simulink library "Electrical_to_Mechanical_gen"  (R2016a)
settings: Solver=ode45  StartTime=0.0  StopTime=10.0  RelTol=1e-3
undefined symbols (not defined in the file): API1dcac_efficiency, API2dcac_efficiency, API3dcac_efficiency, APIdcac_efficiency, aux_power_state, auxEmot_inertia, auxEmot_nTab_3rdD, auxEmot_power, auxEmot_pwrAC, auxEmot_Tau, auxEmot_trqTab_2ndD, auxEmot_vltTab_1stD, AWR_InvStError, DiscIntNeverNeededParam, drvEmot_emot_Cth_rotor, drvEmot_emot_Cth_stator, drvEmot_emot_dtrqEmotNeg, drvEmot_emot_dtrqEmotPtv, drvEmot_emot_inv_pwrLoss, drvEmot_emot_mot_pwrLoss, drvEmot_emot_Rth_rotor_oil, drvEmot_emot_Rth_stator_oil, drvEmot_emot_Rth_stator_rotor, drvEmot_emot_Trotor_init, drvEmot_emot_trqMaxRow, drvEmot_emot_trqMinRow, drvEmot_emot_Tstator_init, drvEmot_inv_Cth_cooling_plate, drvEmot_inv_Cth_diode, drvEmot_inv_Cth_IGBT, drvEmot_inv_n_IGBT_per_Switch, drvEmot_inv_Rth_cooling_plate_coolant, drvEmot_inv_Rth_PS_cooling_plate, drvEmot_inv_Tplate_init, drvEmot_inv_Tpowerstack_init, drvEmot_RefTqeMOT, emot_AcCmprFront_inertia, emot_AcCmprFront_nTab_3rdD, emot_AcCmprFront_pwrAC, emot_AcCmprFront_Tau, emot_AcCmprFront_trqTab_2ndD, emot_AcCmprFront_vltTab_1stD, emot_AcCmprRear_inertia, emot_AcCmprRear_nTab_3rdD, emot_AcCmprRear_pwrAC, emot_AcCmprRear_Tau, emot_AcCmprRear_trqTab_2ndD, emot_AcCmprRear_vltTab_1stD, emot_AirCmpr_inertia, emot_AirCmpr_nTab_3rdD, emot_AirCmpr_pwrAC, emot_AirCmpr_Tau, emot_AirCmpr_trqTab_2ndD, emot_AirCmpr_vltTab_1stD, emot_aircomp_power, FirstDrivenAxle_FirstDrivenAxleNoOfEmot, SecondDrivenAxle_SecondDrivenAxleNoOfEmot
libraries: Electrical_to_Mechanical_gen x4, simulink x4
(part 2 of 2)

== system Electrical_to_Mechanical_gen/EDB_DriveEmot/Emot2_3 ==
  hvs_emot_Emot2_angVel : Inport
  voltBatHV2 : Inport  Port=2
  trqEmotDesPhy2 : Inport  Port=3
  emot_CMD2 : Inport  Port=4
  voltBatHV3 : Inport  Port=5
  trqEmotDesPhy3 : Inport  Port=6
  emot_CMD3 : Inport  Port=7
  hvs_drvEmot2Oil_Temperature : Inport  Port=8
  inv_coolant_temperature : Inport  Port=9
  Emot2_Selection : Inport  Port=10
  Emot3_Selection : Inport  Port=11
  hvs_emot_Emot3_angVel : Inport  Port=12
  hvs_drvEmot3Oil_Temperature : Inport  Port=13
  Bus Creator1 : BusCreator  Inputs=12
  Bus Creator2 : BusCreator  Inputs=12
  Bus Creator3 : BusCreator  Inputs=2
  e-Motor2 : Electrical_to_Mechanical_gen/e-Motor  SystemSampleTime=-1
  e-Motor3 : Electrical_to_Mechanical_gen/e-Motor  SystemSampleTime=-1
  emot2_3B : Outport
  wires:
  e-Motor3/12 -> Bus Creator2/12
  e-Motor3/11 -> Bus Creator2/11
  e-Motor2/12 -> Bus Creator1/12
  e-Motor2/11 -> Bus Creator1/11
  e-Motor3/10 -> Bus Creator2/10
  e-Motor2/10 -> Bus Creator1/10
  hvs_drvEmot3Oil_Temperature/1 -> e-Motor3/5
  Emot3_Selection/1 -> e-Motor3/Enable
  Emot2_Selection/1 -> e-Motor2/Enable
  emot_CMD3/1 -> e-Motor3/4
  emot_CMD2/1 -> e-Motor2/4
  e-Motor3/5 -> Bus Creator2/5
  e-Motor3/4 -> Bus Creator2/4
  e-Motor3/3 -> Bus Creator2/3
  e-Motor3/2 -> Bus Creator2/2
  e-Motor3/1 -> Bus Creator2/1
  e-Motor2/5 -> Bus Creator1/5
  e-Motor2/2 -> Bus Creator1/2
  e-Motor2/1 -> Bus Creator1/1
  e-Motor2/4 -> Bus Creator1/4
  e-Motor2/3 -> Bus Creator1/3
  hvs_emot_Emot2_angVel/1 -> e-Motor2/1
  trqEmotDesPhy2/1 -> e-Motor2/3
  voltBatHV2/1 -> e-Motor2/2
  hvs_emot_Emot3_angVel/1 -> e-Motor3/1
  voltBatHV3/1 -> e-Motor3/2
  Bus Creator1/1 -> Bus Creator3/1  "emot2B"
  Bus Creator2/1 -> Bus Creator3/2  "emot3B"
  trqEmotDesPhy3/1 -> e-Motor3/3
  Bus Creator3/1 -> emot2_3B/1  "emot2_3B"
  hvs_drvEmot2Oil_Temperature/1 -> e-Motor2/5
  inv_coolant_temperature/1 -> e-Motor3/6, e-Motor2/6
  e-Motor3/7 -> Bus Creator2/7
  e-Motor3/6 -> Bus Creator2/6
  e-Motor3/8 -> Bus Creator2/8
  e-Motor3/9 -> Bus Creator2/9
  e-Motor2/6 -> Bus Creator1/6
  e-Motor2/7 -> Bus Creator1/7
  e-Motor2/9 -> Bus Creator1/9
  e-Motor2/8 -> Bus Creator1/8

== system Electrical_to_Mechanical_gen/EDB_DriveEmot/MotorSelection ==
  MidAxle : Constant  Value=FirstDrivenAxle_FirstDrivenAxleNoOfEmot
  RearAxle : Constant  Value=SecondDrivenAxle_SecondDrivenAxleNoOfEmot
  Truth Table : Truth Table  TreatAsAtomicUnit=on
  Emot1_Selection : Outport
  Emot2_Selection : Outport  Port=2
  Emot3_Selection : Outport  Port=3
  Emot4_Selection : Outport  Port=4
  wires:
  Truth Table/4(y4) -> Emot4_Selection/1
  Truth Table/3(y3) -> Emot3_Selection/1
  Truth Table/2(y2) -> Emot2_Selection/1
  Truth Table/1(y1) -> Emot1_Selection/1
  RearAxle/1 -> Truth Table/2(u2)
  MidAxle/1 -> Truth Table/1(u1)

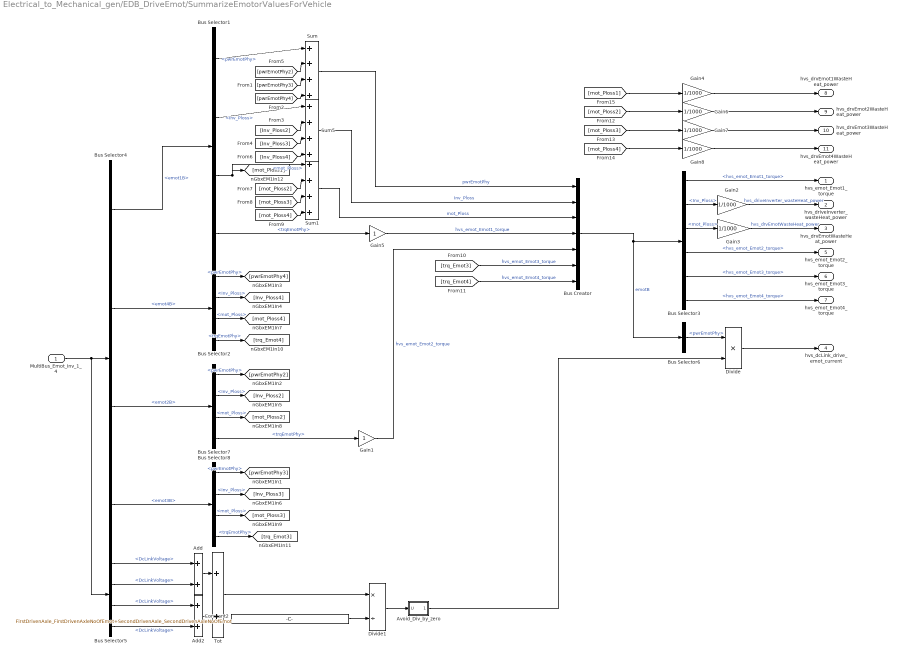
== system Electrical_to_Mechanical_gen/EDB_DriveEmot/SummarizeEmotorValuesForVehicle ==
  MultiBus_Emot_Inv_1_4 : Inport
  Add : Sum
  Add2 : Sum
  Avoid_Div_by_zero : Subsystem
  Bus Creator : BusCreator  Inputs=7
  Bus Selector{1..2,7..8} (4 alike) : BusSelector  OutputSignals=pwrEmotPhy,Inv_Ploss,mot_Ploss,trqEmotPhy
  Bus Selector3 : BusSelector  OutputSignals=hvs_emot_Emot1_torque,Inv_Ploss,mot_Ploss,hvs_emot_Emot2_torque,hvs_emot_Emot3_torque,hvs_emot_Emot4_torque
  Bus Selector4 : BusSelector  OutputSignals=emot1_4B.emot1B,emot1_4B.emot4B,emot2_3B.emot2B,emot2_3B.emot3B
  Bus Selector5 : BusSelector  OutputSignals=emot1_4B.emot1B.DcLinkVoltage,emot1_4B.emot4B.DcLinkVoltage,emot2_3B.emot2B.DcLinkVoltage,emot2_3B.emot3B.DcLinkVoltage
  Bus Selector6 : BusSelector  OutputSignals=pwrEmotPhy
  Constant2 : Constant  Value=FirstDrivenAxle_FirstDrivenAxleNoOfEmot+SecondDrivenAxle_SecondDrivenAxleNoOfEmot
  Divide : Product  Inputs=**
  Divide1 : Product  Inputs=*/
  Gain1 : Gain
  Gain{2..4,6..8} (6 alike) : Gain  Gain=1/1000
  Gain5 : Gain
  Sum : Sum  Inputs=|++++
  Sum1 : Sum  Inputs=|++++
  Sum5 : Sum  Inputs=|++++
  Tot : Sum
  hvs_emot_Emot1_torque : Outport
  hvs_driveInverter_wasteHeat_power : Outport  Port=2
  hvs_drvEmotWasteHeat_power : Outport  Port=3
  hvs_dcLink_drive_emot_current : Outport  Port=4
  hvs_emot_Emot2_torque : Outport  Port=5
  hvs_emot_Emot3_torque : Outport  Port=6
  hvs_emot_Emot4_torque : Outport  Port=7
  hvs_drvEmot1WasteHeat_power : Outport  Port=8
  hvs_drvEmot2WasteHeat_power : Outport  Port=9
  hvs_drvEmot3WasteHeat_power : Outport  Port=10
  hvs_drvEmot4WasteHeat_power : Outport  Port=11
  wires:
  Gain8/1 -> hvs_drvEmot4WasteHeat_power/1
  Gain7/1 -> hvs_drvEmot3WasteHeat_power/1
  Gain6/1 -> hvs_drvEmot2WasteHeat_power/1
  Gain4/1 -> hvs_drvEmot1WasteHeat_power/1
  [mot_Ploss4] -> Gain8/1
  [mot_Ploss3] -> Gain7/1
  [mot_Ploss2] -> Gain6/1
  [mot_Ploss1] -> Gain4/1
  Bus Selector3/6 -> hvs_emot_Emot4_torque/1  "<hvs_emot_Emot4_torque>"
  Bus Selector3/5 -> hvs_emot_Emot3_torque/1  "<hvs_emot_Emot3_torque>"
  Bus Selector3/4 -> hvs_emot_Emot2_torque/1  "<hvs_emot_Emot2_torque>"
  Bus Selector3/1 -> hvs_emot_Emot1_torque/1  "<hvs_emot_Emot1_torque>"
  [trq_Emot4] -> Bus Creator/7  "hvs_emot_Emot4_torque"
  [trq_Emot3] -> Bus Creator/6  "hvs_emot_Emot3_torque"
  Bus Selector2/4 -> [trq_Emot4]  "<trqEmotPhy>"
  Tot/1 -> Divide1/1
  Constant2/1 -> Divide1/2
  Add2/1 -> Tot/2
  Bus Selector5/4 -> Add2/2  "<DcLinkVoltage>"
  Bus Selector5/3 -> Add2/1  "<DcLinkVoltage>"
  Gain1/1 -> Bus Creator/5  "hvs_emot_Emot2_torque"
  Bus Selector8/4 -> [trq_Emot3]  "<trqEmotPhy>"
  Bus Selector7/4 -> Gain1/1  "<trqEmotPhy>"
  [mot_Ploss4] -> Sum1/4
  [mot_Ploss3] -> Sum1/3
  [mot_Ploss2] -> Sum1/2
  Bus Selector8/3 -> [mot_Ploss3]  "<mot_Ploss>"
  Bus Selector7/3 -> [mot_Ploss2]  "<mot_Ploss>"
  Bus Selector8/2 -> [Inv_Ploss3]  "<Inv_Ploss>"
  Bus Selector7/2 -> [Inv_Ploss2]  "<Inv_Ploss>"
  [Inv_Ploss4] -> Sum5/4
  [Inv_Ploss3] -> Sum5/3
  [Inv_Ploss2] -> Sum5/2
  [pwrEmotPhy4] -> Sum/4
  [pwrEmotPhy3] -> Sum/3
  [pwrEmotPhy2] -> Sum/2
  Bus Selector2/1 -> [pwrEmotPhy4]  "<pwrEmotPhy>"
  Bus Selector8/1 -> [pwrEmotPhy3]  "<pwrEmotPhy>"
  Bus Selector7/1 -> [pwrEmotPhy2]  "<pwrEmotPhy>"
  Bus Selector4/3 -> Bus Selector7/1  "<emot2B>"
  Bus Selector4/4 -> Bus Selector8/1  "<emot3B>"
  Gain3/1 -> hvs_drvEmotWasteHeat_power/1  "hvs_drvEmotWasteHeat_power"
  Bus Selector3/3 -> Gain3/1  "<mot_Ploss>"
  Gain2/1 -> hvs_driveInverter_wasteHeat_power/1  "hvs_driveInverter_wasteHeat_power"
  Bus Selector3/2 -> Gain2/1  "<Inv_Ploss>"
  Divide/1 -> hvs_dcLink_drive_emot_current/1
  Avoid_Div_by_zero/1(1/U) -> Divide/2
  Bus Selector6/1 -> Divide/1  "<pwrEmotPhy>"
  Divide1/1 -> Avoid_Div_by_zero/1(U)
  Add/1 -> Tot/1
  Bus Selector5/2 -> Add/2  "<DcLinkVoltage>"
  Bus Selector5/1 -> Add/1  "<DcLinkVoltage>"
  Bus Creator/1 -> Bus Selector6/1, Bus Selector3/1  "emotB"
  MultiBus_Emot_Inv_1_4/1 -> Bus Selector4/1, Bus Selector5/1
  Bus Selector4/1 -> Bus Selector1/1  "<emot1B>"
  Bus Selector4/2 -> Bus Selector2/1  "<emot4B>"
  Bus Selector1/1 -> Sum/1  "<pwrEmotPhy>"
  Bus Selector1/2 -> Sum5/1  "<Inv_Ploss>"
  Bus Selector2/2 -> [Inv_Ploss4]  "<Inv_Ploss>"
  Bus Selector1/3 -> Sum1/1, [mot_Ploss1]  "<mot_Ploss>"
  Bus Selector2/3 -> [mot_Ploss4]  "<mot_Ploss>"
  Bus Selector1/4 -> Gain5/1  "<trqEmotPhy>"
  Sum/1 -> Bus Creator/1  "pwrEmotPhy"
  Sum5/1 -> Bus Creator/2  "Inv_Ploss"
  Sum1/1 -> Bus Creator/3  "mot_Ploss"
  Gain5/1 -> Bus Creator/4  "hvs_emot_Emot1_torque"

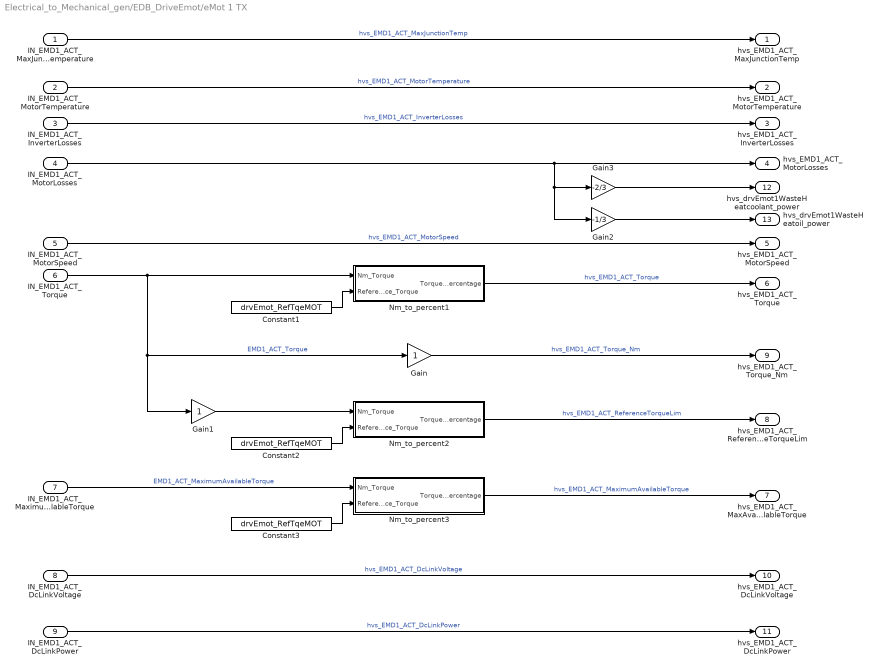
== system Electrical_to_Mechanical_gen/EDB_DriveEmot/eMot 1 TX ==
  IN_EMD1_ACT_MaxJunctionTemperature : Inport
  IN_EMD1_ACT_MotorTemperature : Inport  Port=2
  IN_EMD1_ACT_InverterLosses : Inport  Port=3
  IN_EMD1_ACT_MotorLosses : Inport  Port=4
  IN_EMD1_ACT_MotorSpeed : Inport  Port=5
  IN_EMD1_ACT_Torque : Inport  Port=6
  IN_EMD1_ACT_MaximumAvailableTorque : Inport  Port=7
  IN_EMD1_ACT_DcLinkVoltage : Inport  Port=8
  IN_EMD1_ACT_DcLinkPower : Inport  Port=9
  Constant1 : Constant  Value=drvEmot_RefTqeMOT
  Constant2 : Constant  Value=drvEmot_RefTqeMOT
  Constant3 : Constant  Value=drvEmot_RefTqeMOT
  Gain : Gain
  Gain1 : Gain
  Gain2 : Gain  Gain=-1/3
  Gain3 : Gain  Gain=-2/3
  Nm_to_percent1 : Subsystem
  Nm_to_percent2 : Subsystem
  Nm_to_percent3 : Subsystem
  hvs_EMD1_ACT_MaxJunctionTemp : Outport
  hvs_EMD1_ACT_MotorTemperature : Outport  Port=2
  hvs_EMD1_ACT_InverterLosses : Outport  Port=3
  hvs_EMD1_ACT_MotorLosses : Outport  Port=4
  hvs_EMD1_ACT_MotorSpeed : Outport  Port=5
  hvs_EMD1_ACT_Torque : Outport  Port=6
  hvs_EMD1_ACT_MaxAvailableTorque : Outport  Port=7
  hvs_EMD1_ACT_ReferenceTorqueLim : Outport  Port=8
  hvs_EMD1_ACT_Torque_Nm : Outport  Port=9
  hvs_EMD1_ACT_DcLinkVoltage : Outport  Port=10
  hvs_EMD1_ACT_DcLinkPower : Outport  Port=11
  hvs_drvEmot1WasteHeatcoolant_power : Outport  Port=12
  hvs_drvEmot1WasteHeatoil_power : Outport  Port=13
  wires:
  IN_EMD1_ACT_DcLinkVoltage/1 -> hvs_EMD1_ACT_DcLinkVoltage/1  "hvs_EMD1_ACT_DcLinkVoltage"
  IN_EMD1_ACT_DcLinkPower/1 -> hvs_EMD1_ACT_DcLinkPower/1  "hvs_EMD1_ACT_DcLinkPower"
  Nm_to_percent2/1(Torque_Percentage) -> hvs_EMD1_ACT_ReferenceTorqueLim/1  "hvs_EMD1_ACT_ReferenceTorqueLim"
  Constant2/1 -> Nm_to_percent2/2(Reference_Torque)
  Gain1/1 -> Nm_to_percent2/1(Nm_Torque)
  Gain/1 -> hvs_EMD1_ACT_Torque_Nm/1  "hvs_EMD1_ACT_Torque_Nm"
  Constant1/1 -> Nm_to_percent1/2(Reference_Torque)
  IN_EMD1_ACT_Torque/1 -> Nm_to_percent1/1(Nm_Torque), Gain1/1, Gain/1  "EMD1_ACT_Torque"
  IN_EMD1_ACT_MaximumAvailableTorque/1 -> Nm_to_percent3/1(Nm_Torque)  "EMD1_ACT_MaximumAvailableTorque"
  Constant3/1 -> Nm_to_percent3/2(Reference_Torque)
  Nm_to_percent1/1(Torque_Percentage) -> hvs_EMD1_ACT_Torque/1  "hvs_EMD1_ACT_Torque"
  Nm_to_percent3/1(Torque_Percentage) -> hvs_EMD1_ACT_MaxAvailableTorque/1  "hvs_EMD1_ACT_MaximumAvailableTorque"
  IN_EMD1_ACT_InverterLosses/1 -> hvs_EMD1_ACT_InverterLosses/1  "hvs_EMD1_ACT_InverterLosses"
  IN_EMD1_ACT_MotorTemperature/1 -> hvs_EMD1_ACT_MotorTemperature/1  "hvs_EMD1_ACT_MotorTemperature"
  IN_EMD1_ACT_MaxJunctionTemperature/1 -> hvs_EMD1_ACT_MaxJunctionTemp/1  "hvs_EMD1_ACT_MaxJunctionTemp"
  IN_EMD1_ACT_MotorSpeed/1 -> hvs_EMD1_ACT_MotorSpeed/1  "hvs_EMD1_ACT_MotorSpeed"
  IN_EMD1_ACT_MotorLosses/1 -> Gain3/1, Gain2/1, hvs_EMD1_ACT_MotorLosses/1
  Gain2/1 -> hvs_drvEmot1WasteHeatoil_power/1
  Gain3/1 -> hvs_drvEmot1WasteHeatcoolant_power/1

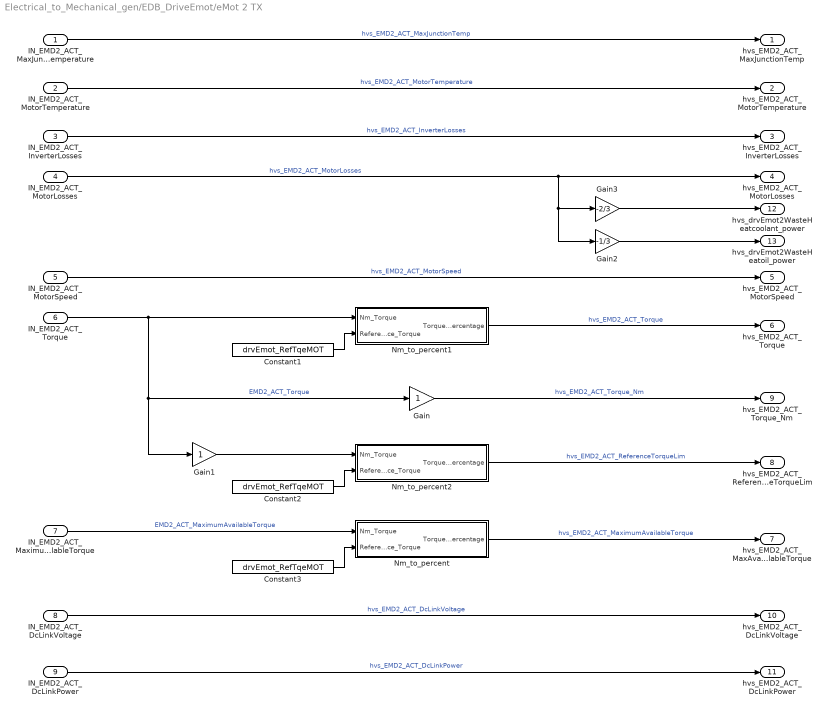
== system Electrical_to_Mechanical_gen/EDB_DriveEmot/eMot 2 TX ==
  IN_EMD2_ACT_MaxJunctionTemperature : Inport
  IN_EMD2_ACT_MotorTemperature : Inport  Port=2
  IN_EMD2_ACT_InverterLosses : Inport  Port=3
  IN_EMD2_ACT_MotorLosses : Inport  Port=4
  IN_EMD2_ACT_MotorSpeed : Inport  Port=5
  IN_EMD2_ACT_Torque : Inport  Port=6
  IN_EMD2_ACT_MaximumAvailableTorque : Inport  Port=7
  IN_EMD2_ACT_DcLinkVoltage : Inport  Port=8
  IN_EMD2_ACT_DcLinkPower : Inport  Port=9
  Constant1 : Constant  Value=drvEmot_RefTqeMOT
  Constant2 : Constant  Value=drvEmot_RefTqeMOT
  Constant3 : Constant  Value=drvEmot_RefTqeMOT
  Gain : Gain
  Gain1 : Gain
  Gain2 : Gain  Gain=-1/3
  Gain3 : Gain  Gain=-2/3
  Nm_to_percent : Subsystem
  Nm_to_percent1 : Subsystem
  Nm_to_percent2 : Subsystem
  hvs_EMD2_ACT_MaxJunctionTemp : Outport
  hvs_EMD2_ACT_MotorTemperature : Outport  Port=2
  hvs_EMD2_ACT_InverterLosses : Outport  Port=3
  hvs_EMD2_ACT_MotorLosses : Outport  Port=4
  hvs_EMD2_ACT_MotorSpeed : Outport  Port=5
  hvs_EMD2_ACT_Torque : Outport  Port=6
  hvs_EMD2_ACT_MaxAvailableTorque : Outport  Port=7
  hvs_EMD2_ACT_ReferenceTorqueLim : Outport  Port=8
  hvs_EMD2_ACT_Torque_Nm : Outport  Port=9
  hvs_EMD2_ACT_DcLinkVoltage : Outport  Port=10
  hvs_EMD2_ACT_DcLinkPower : Outport  Port=11
  hvs_drvEmot2WasteHeatcoolant_power : Outport  Port=12
  hvs_drvEmot2WasteHeatoil_power : Outport  Port=13
  wires:
  IN_EMD2_ACT_DcLinkPower/1 -> hvs_EMD2_ACT_DcLinkPower/1  "hvs_EMD2_ACT_DcLinkPower"
  IN_EMD2_ACT_DcLinkVoltage/1 -> hvs_EMD2_ACT_DcLinkVoltage/1  "hvs_EMD2_ACT_DcLinkVoltage"
  Nm_to_percent2/1(Torque_Percentage) -> hvs_EMD2_ACT_ReferenceTorqueLim/1  "hvs_EMD2_ACT_ReferenceTorqueLim"
  Constant2/1 -> Nm_to_percent2/2(Reference_Torque)
  Gain1/1 -> Nm_to_percent2/1(Nm_Torque)
  Gain/1 -> hvs_EMD2_ACT_Torque_Nm/1  "hvs_EMD2_ACT_Torque_Nm"
  Constant1/1 -> Nm_to_percent1/2(Reference_Torque)
  IN_EMD2_ACT_Torque/1 -> Nm_to_percent1/1(Nm_Torque), Gain1/1, Gain/1  "EMD2_ACT_Torque"
  IN_EMD2_ACT_MaximumAvailableTorque/1 -> Nm_to_percent/1(Nm_Torque)  "EMD2_ACT_MaximumAvailableTorque"
  Constant3/1 -> Nm_to_percent/2(Reference_Torque)
  IN_EMD2_ACT_MotorLosses/1 -> Gain3/1, Gain2/1, hvs_EMD2_ACT_MotorLosses/1  "hvs_EMD2_ACT_MotorLosses"
  IN_EMD2_ACT_InverterLosses/1 -> hvs_EMD2_ACT_InverterLosses/1  "hvs_EMD2_ACT_InverterLosses"
  IN_EMD2_ACT_MotorTemperature/1 -> hvs_EMD2_ACT_MotorTemperature/1  "hvs_EMD2_ACT_MotorTemperature"
  IN_EMD2_ACT_MaxJunctionTemperature/1 -> hvs_EMD2_ACT_MaxJunctionTemp/1  "hvs_EMD2_ACT_MaxJunctionTemp"
  IN_EMD2_ACT_MotorSpeed/1 -> hvs_EMD2_ACT_MotorSpeed/1  "hvs_EMD2_ACT_MotorSpeed"
  Nm_to_percent1/1(Torque_Percentage) -> hvs_EMD2_ACT_Torque/1  "hvs_EMD2_ACT_Torque"
  Nm_to_percent/1(Torque_Percentage) -> hvs_EMD2_ACT_MaxAvailableTorque/1  "hvs_EMD2_ACT_MaximumAvailableTorque"
  Gain2/1 -> hvs_drvEmot2WasteHeatoil_power/1
  Gain3/1 -> hvs_drvEmot2WasteHeatcoolant_power/1

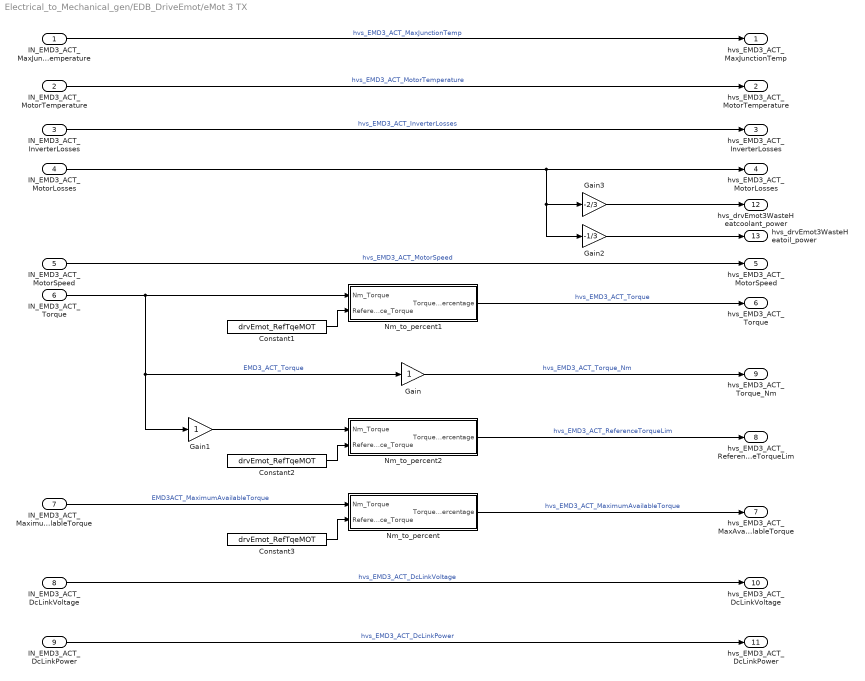
== system Electrical_to_Mechanical_gen/EDB_DriveEmot/eMot 3 TX ==
  IN_EMD3_ACT_MaxJunctionTemperature : Inport
  IN_EMD3_ACT_MotorTemperature : Inport  Port=2
  IN_EMD3_ACT_InverterLosses : Inport  Port=3
  IN_EMD3_ACT_MotorLosses : Inport  Port=4
  IN_EMD3_ACT_MotorSpeed : Inport  Port=5
  IN_EMD3_ACT_Torque : Inport  Port=6
  IN_EMD3_ACT_MaximumAvailableTorque : Inport  Port=7
  IN_EMD3_ACT_DcLinkVoltage : Inport  Port=8
  IN_EMD3_ACT_DcLinkPower : Inport  Port=9
  Constant1 : Constant  Value=drvEmot_RefTqeMOT
  Constant2 : Constant  Value=drvEmot_RefTqeMOT
  Constant3 : Constant  Value=drvEmot_RefTqeMOT
  Gain : Gain
  Gain1 : Gain
  Gain2 : Gain  Gain=-1/3
  Gain3 : Gain  Gain=-2/3
  Nm_to_percent : Subsystem
  Nm_to_percent1 : Subsystem
  Nm_to_percent2 : Subsystem
  hvs_EMD3_ACT_MaxJunctionTemp : Outport
  hvs_EMD3_ACT_MotorTemperature : Outport  Port=2
  hvs_EMD3_ACT_InverterLosses : Outport  Port=3
  hvs_EMD3_ACT_MotorLosses : Outport  Port=4
  hvs_EMD3_ACT_MotorSpeed : Outport  Port=5
  hvs_EMD3_ACT_Torque : Outport  Port=6
  hvs_EMD3_ACT_MaxAvailableTorque : Outport  Port=7
  hvs_EMD3_ACT_ReferenceTorqueLim : Outport  Port=8
  hvs_EMD3_ACT_Torque_Nm : Outport  Port=9
  hvs_EMD3_ACT_DcLinkVoltage : Outport  Port=10
  hvs_EMD3_ACT_DcLinkPower : Outport  Port=11
  hvs_drvEmot3WasteHeatcoolant_power : Outport  Port=12
  hvs_drvEmot3WasteHeatoil_power : Outport  Port=13
  wires:
  IN_EMD3_ACT_DcLinkPower/1 -> hvs_EMD3_ACT_DcLinkPower/1  "hvs_EMD3_ACT_DcLinkPower"
  IN_EMD3_ACT_DcLinkVoltage/1 -> hvs_EMD3_ACT_DcLinkVoltage/1  "hvs_EMD3_ACT_DcLinkVoltage"
  Nm_to_percent2/1(Torque_Percentage) -> hvs_EMD3_ACT_ReferenceTorqueLim/1  "hvs_EMD3_ACT_ReferenceTorqueLim"
  Constant2/1 -> Nm_to_percent2/2(Reference_Torque)
  Gain1/1 -> Nm_to_percent2/1(Nm_Torque)
  Gain/1 -> hvs_EMD3_ACT_Torque_Nm/1  "hvs_EMD3_ACT_Torque_Nm"
  Constant1/1 -> Nm_to_percent1/2(Reference_Torque)
  IN_EMD3_ACT_Torque/1 -> Nm_to_percent1/1(Nm_Torque), Gain1/1, Gain/1  "EMD3_ACT_Torque"
  IN_EMD3_ACT_MaximumAvailableTorque/1 -> Nm_to_percent/1(Nm_Torque)  "EMD3ACT_MaximumAvailableTorque"
  Constant3/1 -> Nm_to_percent/2(Reference_Torque)
  Nm_to_percent1/1(Torque_Percentage) -> hvs_EMD3_ACT_Torque/1  "hvs_EMD3_ACT_Torque"
  Nm_to_percent/1(Torque_Percentage) -> hvs_EMD3_ACT_MaxAvailableTorque/1  "hvs_EMD3_ACT_MaximumAvailableTorque"
  IN_EMD3_ACT_InverterLosses/1 -> hvs_EMD3_ACT_InverterLosses/1  "hvs_EMD3_ACT_InverterLosses"
  IN_EMD3_ACT_MaxJunctionTemperature/1 -> hvs_EMD3_ACT_MaxJunctionTemp/1  "hvs_EMD3_ACT_MaxJunctionTemp"
  IN_EMD3_ACT_MotorTemperature/1 -> hvs_EMD3_ACT_MotorTemperature/1  "hvs_EMD3_ACT_MotorTemperature"
  IN_EMD3_ACT_MotorSpeed/1 -> hvs_EMD3_ACT_MotorSpeed/1  "hvs_EMD3_ACT_MotorSpeed"
  IN_EMD3_ACT_MotorLosses/1 -> hvs_EMD3_ACT_MotorLosses/1, Gain3/1, Gain2/1
  Gain2/1 -> hvs_drvEmot3WasteHeatoil_power/1
  Gain3/1 -> hvs_drvEmot3WasteHeatcoolant_power/1

== system Electrical_to_Mechanical_gen/EDB_DriveEmot/eMot 4 TX ==
  IN_EMD4_ACT_MaxJunctionTemperature : Inport
  IN_EMD4_ACT_MotorTemperature : Inport  Port=2
  IN_EMD4_ACT_InverterLosses : Inport  Port=3
  IN_EMD4_ACT_MotorLosses : Inport  Port=4
  IN_EMD4_ACT_MotorSpeed : Inport  Port=5
  IN_EMD4_ACT_Torque : Inport  Port=6
  IN_EMD4_ACT_MaximumAvailableTorque : Inport  Port=7
  IN_EMD4_ACT_DcLinkVoltage : Inport  Port=8
  IN_EMD4_ACT_DcLinkPower : Inport  Port=9
  Constant1 : Constant  Value=drvEmot_RefTqeMOT
  Constant2 : Constant  Value=drvEmot_RefTqeMOT
  Constant3 : Constant  Value=drvEmot_RefTqeMOT
  Gain : Gain
  Gain1 : Gain
  Gain2 : Gain  Gain=-1/3
  Gain3 : Gain  Gain=-2/3
  Nm_to_percent1 : Subsystem
  Nm_to_percent2 : Subsystem
  Nm_to_percent3 : Subsystem
  hvs_EMD4_ACT_MaxJunctionTemperature : Outport
  hvs_EMD4_ACT_MotorTemperature : Outport  Port=2
  hvs_EMD4_ACT_InverterLosses : Outport  Port=3
  hvs_EMD4_ACT_MotorLosses : Outport  Port=4
  hvs_EMD4_ACT_MotorSpeed : Outport  Port=5
  hvs_EMD4_ACT_Torque : Outport  Port=6
  hvs_EMD4_ACT_MaxAvailableTorque : Outport  Port=7
  hvs_EMD4_ACT_ReferenceTorqueLim : Outport  Port=8
  hvs_EMD4_ACT_Torque_Nm : Outport  Port=9
  hvs_EMD4_ACT_DcLinkVoltage : Outport  Port=10
  hvs_EMD4_ACT_DcLinkPower : Outport  Port=11
  hvs_drvEmot4WasteHeatcoolant_power : Outport  Port=12
  hvs_drvEmot4WasteHeatoil_power : Outport  Port=13
  wires:
  IN_EMD4_ACT_DcLinkPower/1 -> hvs_EMD4_ACT_DcLinkPower/1  "IN_EMD4_ACT_DcLinkPower"
  IN_EMD4_ACT_DcLinkVoltage/1 -> hvs_EMD4_ACT_DcLinkVoltage/1  "hvs_EMD4_ACT_DcLinkVoltage"
  Nm_to_percent2/1(Torque_Percentage) -> hvs_EMD4_ACT_ReferenceTorqueLim/1  "hvs_EMD4_ACT_ReferenceTorqueLim"
  Constant2/1 -> Nm_to_percent2/2(Reference_Torque)
  Gain1/1 -> Nm_to_percent2/1(Nm_Torque)
  Gain/1 -> hvs_EMD4_ACT_Torque_Nm/1  "hvs_EMD4_ACT_Torque_Nm"
  Constant1/1 -> Nm_to_percent1/2(Reference_Torque)
  IN_EMD4_ACT_Torque/1 -> Nm_to_percent1/1(Nm_Torque), Gain1/1, Gain/1  "EMD4_ACT_Torque"
  IN_EMD4_ACT_MaximumAvailableTorque/1 -> Nm_to_percent3/1(Nm_Torque)  "EMD4_ACT_MaximumAvailableTorque"
  Constant3/1 -> Nm_to_percent3/2(Reference_Torque)
  Nm_to_percent1/1(Torque_Percentage) -> hvs_EMD4_ACT_Torque/1  "hvs_EMD4_ACT_Torque"
  Nm_to_percent3/1(Torque_Percentage) -> hvs_EMD4_ACT_MaxAvailableTorque/1  "hvs_EMD4_ACT_MaximumAvailableTorque"
  IN_EMD4_ACT_InverterLosses/1 -> hvs_EMD4_ACT_InverterLosses/1  "hvs_EMD4_ACT_InverterLosses"
  IN_EMD4_ACT_MotorTemperature/1 -> hvs_EMD4_ACT_MotorTemperature/1  "hvs_EMD4_ACT_MotorTemperature"
  IN_EMD4_ACT_MaxJunctionTemperature/1 -> hvs_EMD4_ACT_MaxJunctionTemperature/1  "hvs_EMD4_ACT_MaxJunctionTemperature"
  IN_EMD4_ACT_MotorSpeed/1 -> hvs_EMD4_ACT_MotorSpeed/1  "hvs_EMD4_ACT_MotorSpeed"
  IN_EMD4_ACT_MotorLosses/1 -> Gain3/1, Gain2/1, hvs_EMD4_ACT_MotorLosses/1
  Gain2/1 -> hvs_drvEmot4WasteHeatoil_power/1
  Gain3/1 -> hvs_drvEmot4WasteHeatcoolant_power/1

== system Electrical_to_Mechanical_gen/Emot AC Compressor Front/Avoid_Div_by_zero ==
  U : Inport
  Constant : Constant  Value=10^-6
  Divide : Product  Inputs=/*
  Math Function : Math  Operator=square  SaturateOnIntegerOverflow=on
  Sum : Sum  Inputs=++|
  1/U : Outport
  wires:
  Divide/1 -> 1/U/1
  Math Function/1 -> Divide/1
  Sum/1 -> Divide/2, Math Function/1
  Constant/1 -> Sum/1
  U/1 -> Sum/2

== system Electrical_to_Mechanical_gen/Emot AC Compressor Rear/Avoid_Div_by_zero ==
  U : Inport
  Constant : Constant  Value=10^-6
  Divide : Product  Inputs=/*
  Math Function : Math  Operator=square  SaturateOnIntegerOverflow=on
  Sum : Sum  Inputs=++|
  1/U : Outport
  wires:
  Divide/1 -> 1/U/1
  Math Function/1 -> Divide/1
  Sum/1 -> Divide/2, Math Function/1
  Constant/1 -> Sum/1
  U/1 -> Sum/2

== system Electrical_to_Mechanical_gen/Emot Air Compressor/Avoid_Div_by_zero ==
  U : Inport
  Constant : Constant  Value=10^-6
  Divide : Product  Inputs=/*
  Math Function : Math  Operator=square  SaturateOnIntegerOverflow=on
  Sum : Sum  Inputs=++|
  1/U : Outport
  wires:
  Divide/1 -> 1/U/1
  Math Function/1 -> Divide/1
  Sum/1 -> Divide/2, Math Function/1
  Constant/1 -> Sum/1
  U/1 -> Sum/2

== system Electrical_to_Mechanical_gen/auxEmot/Avoid_Div_by_zero ==
  U : Inport
  Constant : Constant  Value=10^-6
  Divide : Product  Inputs=/*
  Math Function : Math  Operator=square  SaturateOnIntegerOverflow=on
  Sum : Sum  Inputs=++|
  1/U : Outport
  wires:
  U/1 -> Sum/2
  Constant/1 -> Sum/1
  Sum/1 -> Math Function/1, Divide/2
  Math Function/1 -> Divide/1
  Divide/1 -> 1/U/1

== system Electrical_to_Mechanical_gen/e-Motor/Fahrmotoren ==
  nEmot_k : Inport
  nEmot_f : Inport  Port=2
  trqEmot_k : Inport  Port=3
  trqEmot_f : Inport  Port=4
  U_DC_k : Inport  Port=5
  U_DC_f : Inport  Port=6
  mot_Ploss_lookup : Interpolation_n-D  NumberOfTableDimensions=3  Table=drvEmot_emot_mot_pwrLoss  ExtrapMethod=Clip  ValidIndexMayReachLast=on
      settings: InputPortMap=u0,u1,u2,u3,u4,u5
  mot_Ploss : Outport
  wires:
  mot_Ploss_lookup/1 -> mot_Ploss/1
  nEmot_f/1 -> mot_Ploss_lookup/2
  nEmot_k/1 -> mot_Ploss_lookup/1
  trqEmot_k/1 -> mot_Ploss_lookup/3
  trqEmot_f/1 -> mot_Ploss_lookup/4
  U_DC_k/1 -> mot_Ploss_lookup/5
  U_DC_f/1 -> mot_Ploss_lookup/6

== system Electrical_to_Mechanical_gen/e-Motor/Thermic_Model_Inverter ==
  P_WasteHeat_Powerstack : Inport
  T_Coolant : Inport  Port=2
  T_Powerstack : Inport  Port=3
  T_Plate : Inport  Port=4
  Add : Sum  Inputs=+-
  Add1 : Sum  Inputs=+-
  C_IGBT_and_Diode : Subsystem
  C_Plate : Subsystem
  Gain : Gain  Gain=1/drvEmot_inv_n_IGBT_per_Switch
  Gain2 : Gain  Gain=drvEmot_inv_n_IGBT_per_Switch
  R_PS-Plate : Subsystem
  R_Plate-Coolant : Subsystem
  P_Coolant : Outport
  T_Powerstack_new : Outport  Port=2
  T_Plate_new : Outport  Port=3
  wires:
  Add/1 -> C_IGBT_and_Diode/1(P_Heat_eff)
  P_WasteHeat_Powerstack/1 -> Gain/1
  Add1/1 -> C_Plate/1(P_Heat_eff)
  T_Powerstack/1 -> R_PS-Plate/1(T_IGBT), C_IGBT_and_Diode/2(T)
  C_IGBT_and_Diode/1(T_new) -> T_Powerstack_new/1
  T_Plate/1 -> R_Plate-Coolant/1(T_Plate), R_PS-Plate/2(T_Plate), C_Plate/2(T)
  C_Plate/1(T_new) -> T_Plate_new/1
  T_Coolant/1 -> R_Plate-Coolant/2(T_Coolant)
  Gain/1 -> Add/1
  Gain2/1 -> P_Coolant/1
  R_PS-Plate/1(dQ) -> Add/2, Add1/1
  R_Plate-Coolant/1(dQ) -> Add1/2, Gain2/1

== system Electrical_to_Mechanical_gen/e-Motor/Thermic_Model_PMSM_slot2 ==
  P_WasteHeat_Rotor : Inport
  P_WasteHeat_Stator : Inport  Port=2
  T_Oil : Inport  Port=3
  T_Stator : Inport  Port=4
  T_Rotor : Inport  Port=5
  Add : Sum
  Add1 : Sum  Inputs=-+-
  Add2 : Sum  Inputs=++-
  C_Rotor : Subsystem
  C_Stator : Subsystem
  K2degC : Subsystem
  K2degC1 : Subsystem
  R_RotorOil : Subsystem
  R_StatorOil : Subsystem
  R_StatorRotor : Subsystem
  degC2K : Subsystem
  degC2K1 : Subsystem
  degC2K2 : Subsystem
  HeatFlow_eMotor_Oil : Outport
  T_Stator_new : Outport  Port=2
  T_Rotor_new : Outport  Port=3
  wires:
  C_Stator/1(T_new) -> K2degC/1(In1)
  C_Rotor/1(T_new) -> K2degC1/1(In1)
  Add/1 -> HeatFlow_eMotor_Oil/1
  R_StatorOil/1(dQ) -> Add1/1, Add/2
  [A] -> Add/1
  T_Stator/1 -> degC2K1/1(In1)
  P_WasteHeat_Stator/1 -> Add1/2
  Add1/1 -> C_Stator/1(P_Heat_eff)
  R_StatorRotor/1(dQ) -> Add2/1, Add1/3
  T_Rotor/1 -> degC2K2/1(In1)
  R_RotorOil/1(dQ) -> [A], Add2/3
  Add2/1 -> C_Rotor/1(P_Heat_eff)
  P_WasteHeat_Rotor/1 -> Add2/2
  K2degC/1(Out1) -> T_Stator_new/1
  K2degC1/1(Out1) -> T_Rotor_new/1
  T_Oil/1 -> degC2K/1(In1)  "T_Oil"
  degC2K/1(Out1) -> [B], R_StatorOil/1(T_Oil)
  degC2K1/1(Out1) -> R_StatorRotor/1(T_Stator), C_Stator/2(T), R_StatorOil/2(T_Stator)
  degC2K2/1(Out1) -> R_RotorOil/1(T_Rotor), C_Rotor/2(T), R_StatorRotor/2(T_Rotor)
  [B] -> R_RotorOil/2(T_Oil)

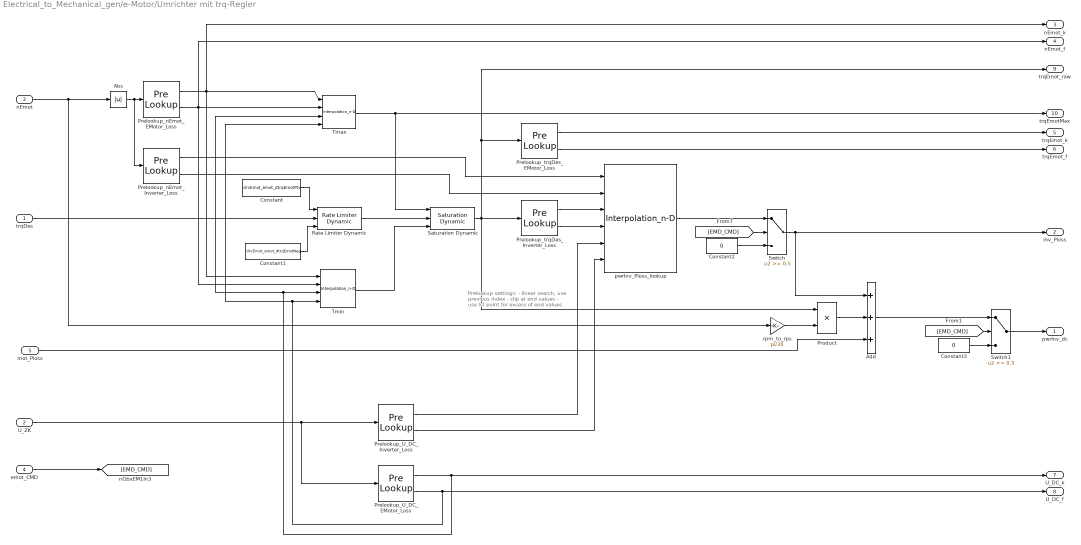
== system Electrical_to_Mechanical_gen/e-Motor/Umrichter mit trq-Regler ==
  note: Prelookup settings:
      | - linear search, use previous index
      | - clip at end values
      | - use lst point for
      | excess of end values
  trqDes : Inport
  U_ZK : Inport  Port=2
  nEmot : Inport  Port=3
  emot_CMD : Inport  Port=4
  mot_Ploss : Inport  Port=5
  Abs : Abs
  Add : Sum  Inputs=+++
  Constant : Constant  Value=drvEmot_emot_dtrqEmotPtv
  Constant1 : Constant  Value=drvEmot_emot_dtrqEmotNeg
  Constant2 : Constant  Value=0
  Constant3 : Constant  Value=0
  Prelookup_U_DC_EMotor_Loss : PreLookup  BreakpointsData=drvEmot_emot_vltTab_3rdD  IndexSearchMethod=Linear search  BeginIndexSearchUsingPreviousIndexResult=on  UseLastBreakpoint=on
  Prelookup_U_DC_Inverter_Loss : PreLookup  BreakpointsData=drvEmot_inv_vltTab_3rdD  IndexSearchMethod=Linear search  BeginIndexSearchUsingPreviousIndexResult=on  UseLastBreakpoint=on
  Prelookup_nEmot_EMotor_Loss : PreLookup  BreakpointsData=drvEmot_emot_nTab_1stD  IndexSearchMethod=Linear search  BeginIndexSearchUsingPreviousIndexResult=on  UseLastBreakpoint=on
  Prelookup_nEmot_Inverter_Loss : PreLookup  BreakpointsData=drvEmot_inv_nTab_1stD  IndexSearchMethod=Linear search  BeginIndexSearchUsingPreviousIndexResult=on  UseLastBreakpoint=on
  Prelookup_trqDes_EMotor_Loss : PreLookup  BreakpointsData=drvEmot_emot_trqTab_2ndD  IndexSearchMethod=Linear search  BeginIndexSearchUsingPreviousIndexResult=on  UseLastBreakpoint=on
  Prelookup_trqDes_Inverter_Loss : PreLookup  BreakpointsData=drvEmot_inv_trqTab_2ndD  IndexSearchMethod=Linear search  BeginIndexSearchUsingPreviousIndexResult=on  UseLastBreakpoint=on
  Product : Product  RndMeth=Zero
  Rate Limiter Dynamic : simulink/Discontinuities/Rate Limiter Dynamic
  Saturation Dynamic : simulink/Discontinuities/Saturation Dynamic  OutMin=[]  OutMax=[]  OutDataTypeStr=Inherit: Same as second input  OutDataType=fixdt(1, 16)  OutScaling=2^-10  DoSatur=off
  Switch : Switch  Threshold=0.5
  Switch1 : Switch  Threshold=0.5
  Tmax : Interpolation_n-D  Table=drvEmot_emot_trqMaxRow  ExtrapMethod=Clip  ValidIndexMayReachLast=on
  Tmin : Interpolation_n-D  Table=drvEmot_emot_trqMinRow  ExtrapMethod=Clip  ValidIndexMayReachLast=on
  pwrInv_Ploss_lookup : Interpolation_n-D  NumberOfTableDimensions=3  Table=drvEmot_emot_inv_pwrLoss  ExtrapMethod=Clip  ValidIndexMayReachLast=on
      settings: InputPortMap=u0,u1,u2,u3,u4,u5
  rpm_to_rps : Gain  Gain=pi/30
  pwrInv_dc : Outport
  inv_Ploss : Outport  Port=2
  nEmot_k : Outport  Port=3
  nEmot_f : Outport  Port=4
  trqEmot_k : Outport  Port=5
  trqEmot_f : Outport  Port=6
  U_DC_k : Outport  Port=7
  U_DC_f : Outport  Port=8
  trqEmot_raw : Outport  Port=9
  trqEmotMax : Outport  Port=10
  wires:
  Prelookup_trqDes_Inverter_Loss/2 -> pwrInv_Ploss_lookup/4
  Prelookup_trqDes_Inverter_Loss/1 -> pwrInv_Ploss_lookup/3
  Switch/1 -> Add/1, inv_Ploss/1
  Saturation Dynamic/1 -> trqEmot_raw/1, Prelookup_trqDes_EMotor_Loss/1, Product/1, Prelookup_trqDes_Inverter_Loss/1
  Product/1 -> Add/2
  rpm_to_rps/1 -> Product/2
  mot_Ploss/1 -> Add/3
  Constant3/1 -> Switch1/3
  [EMD_CMD] -> Switch1/2
  Add/1 -> Switch1/1
  Constant2/1 -> Switch/3
  [EMD_CMD] -> Switch/2
  emot_CMD/1 -> [EMD_CMD]
  pwrInv_Ploss_lookup/1 -> Switch/1
  Switch1/1 -> pwrInv_dc/1
  Rate Limiter Dynamic/1 -> Saturation Dynamic/2
  Constant1/1 -> Rate Limiter Dynamic/3
  Constant/1 -> Rate Limiter Dynamic/1
  nEmot/1 -> Abs/1, rpm_to_rps/1
  Tmax/1 -> Saturation Dynamic/1, trqEmotMax/1
  Tmin/1 -> Saturation Dynamic/3
  U_ZK/1 -> Prelookup_U_DC_EMotor_Loss/1, Prelookup_U_DC_Inverter_Loss/1
  Prelookup_U_DC_Inverter_Loss/2 -> pwrInv_Ploss_lookup/6
  Prelookup_U_DC_Inverter_Loss/1 -> pwrInv_Ploss_lookup/5
  Prelookup_nEmot_EMotor_Loss/2 -> nEmot_f/1, Tmax/2, Tmin/2
  Prelookup_nEmot_EMotor_Loss/1 -> nEmot_k/1, Tmin/1, Tmax/1
  trqDes/1 -> Rate Limiter Dynamic/2
  Abs/1 -> Prelookup_nEmot_EMotor_Loss/1, Prelookup_nEmot_Inverter_Loss/1
  Prelookup_trqDes_EMotor_Loss/1 -> trqEmot_k/1
  Prelookup_trqDes_EMotor_Loss/2 -> trqEmot_f/1
  Prelookup_U_DC_EMotor_Loss/1 -> Tmin/3, Tmax/3, U_DC_k/1
  Prelookup_U_DC_EMotor_Loss/2 -> U_DC_f/1, Tmin/4, Tmax/4
  Prelookup_nEmot_Inverter_Loss/1 -> pwrInv_Ploss_lookup/1
  Prelookup_nEmot_Inverter_Loss/2 -> pwrInv_Ploss_lookup/2

== system Electrical_to_Mechanical_gen/e-Motor/updatePortNames ==

== system Electrical_to_Mechanical_gen/EDB_DriveEmot/EMD1_Selection/percent_to_Nm2 ==
  Percentage_Torque : Inport
  Reference_Torque : Inport  Port=2
  Constant : Constant  Value=100
  Divide : Product  Inputs=*/
  Product : Product  RndMeth=Zero
  Torque_Nm : Outport
  wires:
  Constant/1 -> Divide/2
  Product/1 -> Divide/1
  Reference_Torque/1 -> Product/2  "Reference_Torque"
  Divide/1 -> Torque_Nm/1  "Torque_Nm"
  Percentage_Torque/1 -> Product/1  "Percentage_Torque"

== system Electrical_to_Mechanical_gen/EDB_DriveEmot/EMD2_Selection/percent_to_Nm2 ==
  Percentage_Torque : Inport
  Reference_Torque : Inport  Port=2
  Constant : Constant  Value=100
  Divide : Product  Inputs=*/
  Product : Product  RndMeth=Zero
  Torque_Nm : Outport
  wires:
  Constant/1 -> Divide/2
  Product/1 -> Divide/1
  Reference_Torque/1 -> Product/2  "Reference_Torque"
  Divide/1 -> Torque_Nm/1  "Torque_Nm"
  Percentage_Torque/1 -> Product/1  "Percentage_Torque"

== system Electrical_to_Mechanical_gen/EDB_DriveEmot/EMD3_Selection/percent_to_Nm2 ==
  Percentage_Torque : Inport
  Reference_Torque : Inport  Port=2
  Constant : Constant  Value=100
  Divide : Product  Inputs=*/
  Product : Product  RndMeth=Zero
  Torque_Nm : Outport
  wires:
  Percentage_Torque/1 -> Product/1  "Percentage_Torque"
  Divide/1 -> Torque_Nm/1  "Torque_Nm"
  Reference_Torque/1 -> Product/2  "Reference_Torque"
  Product/1 -> Divide/1
  Constant/1 -> Divide/2

== system Electrical_to_Mechanical_gen/EDB_DriveEmot/EMD4_Selection/percent_to_Nm2 ==
  Percentage_Torque : Inport
  Reference_Torque : Inport  Port=2
  Constant : Constant  Value=100
  Divide : Product  Inputs=*/
  Product : Product  RndMeth=Zero
  Torque_Nm : Outport
  wires:
  Percentage_Torque/1 -> Product/1  "Percentage_Torque"
  Divide/1 -> Torque_Nm/1  "Torque_Nm"
  Reference_Torque/1 -> Product/2  "Reference_Torque"
  Product/1 -> Divide/1
  Constant/1 -> Divide/2

== system Electrical_to_Mechanical_gen/EDB_DriveEmot/SummarizeEmotorValuesForVehicle/Avoid_Div_by_zero ==
  U : Inport
  Constant : Constant  Value=10^-6
  Math Function : Math  Operator=reciprocal  SaturateOnIntegerOverflow=on
  Switch : Switch  Criteria=u2 > Threshold
  1/U : Outport
  wires:
  U/1 -> Math Function/1, Switch/2
  Constant/1 -> Switch/3
  Math Function/1 -> Switch/1
  Switch/1 -> 1/U/1

== system Electrical_to_Mechanical_gen/EDB_DriveEmot/eMot 1 TX/Nm_to_percent1 ==
  Nm_Torque : Inport
  Reference_Torque : Inport  Port=2
  Constant : Constant  Value=100
  Divide1 : Product  Inputs=*/
  Product1 : Product  RndMeth=Zero
  Torque_Percentage : Outport
  wires:
  Nm_Torque/1 -> Divide1/1  "Nm_Torque"
  Product1/1 -> Torque_Percentage/1  "Torque_Percentage"
  Reference_Torque/1 -> Divide1/2  "Reference_Torque"
  Divide1/1 -> Product1/1
  Constant/1 -> Product1/2

== system Electrical_to_Mechanical_gen/EDB_DriveEmot/eMot 1 TX/Nm_to_percent2 ==
  Nm_Torque : Inport
  Reference_Torque : Inport  Port=2
  Constant : Constant  Value=100
  Divide1 : Product  Inputs=*/
  Product1 : Product  RndMeth=Zero
  Torque_Percentage : Outport
  wires:
  Constant/1 -> Product1/2
  Divide1/1 -> Product1/1
  Reference_Torque/1 -> Divide1/2  "Reference_Torque"
  Product1/1 -> Torque_Percentage/1  "Torque_Percentage"
  Nm_Torque/1 -> Divide1/1  "Nm_Torque"

== system Electrical_to_Mechanical_gen/EDB_DriveEmot/eMot 1 TX/Nm_to_percent3 ==
  Nm_Torque : Inport
  Reference_Torque : Inport  Port=2
  Constant : Constant  Value=100
  Divide1 : Product  Inputs=*/
  Product1 : Product  RndMeth=Zero
  Torque_Percentage : Outport
  wires:
  Nm_Torque/1 -> Divide1/1  "Nm_Torque"
  Product1/1 -> Torque_Percentage/1  "Torque_Percentage"
  Reference_Torque/1 -> Divide1/2  "Reference_Torque"
  Divide1/1 -> Product1/1
  Constant/1 -> Product1/2

== system Electrical_to_Mechanical_gen/EDB_DriveEmot/eMot 2 TX/Nm_to_percent ==
  Nm_Torque : Inport
  Reference_Torque : Inport  Port=2
  Constant : Constant  Value=100
  Divide1 : Product  Inputs=*/
  Product1 : Product  RndMeth=Zero
  Torque_Percentage : Outport
  wires:
  Constant/1 -> Product1/2
  Divide1/1 -> Product1/1
  Reference_Torque/1 -> Divide1/2  "Reference_Torque"
  Product1/1 -> Torque_Percentage/1  "Torque_Percentage"
  Nm_Torque/1 -> Divide1/1  "Nm_Torque"

== system Electrical_to_Mechanical_gen/EDB_DriveEmot/eMot 2 TX/Nm_to_percent1 ==
  Nm_Torque : Inport
  Reference_Torque : Inport  Port=2
  Constant : Constant  Value=100
  Divide1 : Product  Inputs=*/
  Product1 : Product  RndMeth=Zero
  Torque_Percentage : Outport
  wires:
  Constant/1 -> Product1/2
  Divide1/1 -> Product1/1
  Reference_Torque/1 -> Divide1/2  "Reference_Torque"
  Product1/1 -> Torque_Percentage/1  "Torque_Percentage"
  Nm_Torque/1 -> Divide1/1  "Nm_Torque"

== system Electrical_to_Mechanical_gen/EDB_DriveEmot/eMot 2 TX/Nm_to_percent2 ==
  Nm_Torque : Inport
  Reference_Torque : Inport  Port=2
  Constant : Constant  Value=100
  Divide1 : Product  Inputs=*/
  Product1 : Product  RndMeth=Zero
  Torque_Percentage : Outport
  wires:
  Nm_Torque/1 -> Divide1/1  "Nm_Torque"
  Product1/1 -> Torque_Percentage/1  "Torque_Percentage"
  Reference_Torque/1 -> Divide1/2  "Reference_Torque"
  Divide1/1 -> Product1/1
  Constant/1 -> Product1/2

== system Electrical_to_Mechanical_gen/EDB_DriveEmot/eMot 3 TX/Nm_to_percent ==
  Nm_Torque : Inport
  Reference_Torque : Inport  Port=2
  Constant : Constant  Value=100
  Divide1 : Product  Inputs=*/
  Product1 : Product  RndMeth=Zero
  Torque_Percentage : Outport
  wires:
  Nm_Torque/1 -> Divide1/1  "Nm_Torque"
  Product1/1 -> Torque_Percentage/1  "Torque_Percentage"
  Reference_Torque/1 -> Divide1/2  "Reference_Torque"
  Divide1/1 -> Product1/1
  Constant/1 -> Product1/2

== system Electrical_to_Mechanical_gen/EDB_DriveEmot/eMot 3 TX/Nm_to_percent1 ==
  Nm_Torque : Inport
  Reference_Torque : Inport  Port=2
  Constant : Constant  Value=100
  Divide1 : Product  Inputs=*/
  Product1 : Product  RndMeth=Zero
  Torque_Percentage : Outport
  wires:
  Nm_Torque/1 -> Divide1/1  "Nm_Torque"
  Product1/1 -> Torque_Percentage/1  "Torque_Percentage"
  Reference_Torque/1 -> Divide1/2  "Reference_Torque"
  Divide1/1 -> Product1/1
  Constant/1 -> Product1/2

== system Electrical_to_Mechanical_gen/EDB_DriveEmot/eMot 3 TX/Nm_to_percent2 ==
  Nm_Torque : Inport
  Reference_Torque : Inport  Port=2
  Constant : Constant  Value=100
  Divide1 : Product  Inputs=*/
  Product1 : Product  RndMeth=Zero
  Torque_Percentage : Outport
  wires:
  Constant/1 -> Product1/2
  Divide1/1 -> Product1/1
  Reference_Torque/1 -> Divide1/2  "Reference_Torque"
  Product1/1 -> Torque_Percentage/1  "Torque_Percentage"
  Nm_Torque/1 -> Divide1/1  "Nm_Torque"

== system Electrical_to_Mechanical_gen/EDB_DriveEmot/eMot 4 TX/Nm_to_percent1 ==
  Nm_Torque : Inport
  Reference_Torque : Inport  Port=2
  Constant : Constant  Value=100
  Divide1 : Product  Inputs=*/
  Product1 : Product  RndMeth=Zero
  Torque_Percentage : Outport
  wires:
  Constant/1 -> Product1/2
  Divide1/1 -> Product1/1
  Reference_Torque/1 -> Divide1/2  "Reference_Torque"
  Product1/1 -> Torque_Percentage/1  "Torque_Percentage"
  Nm_Torque/1 -> Divide1/1  "Nm_Torque"

== system Electrical_to_Mechanical_gen/EDB_DriveEmot/eMot 4 TX/Nm_to_percent2 ==
  Nm_Torque : Inport
  Reference_Torque : Inport  Port=2
  Constant : Constant  Value=100
  Divide1 : Product  Inputs=*/
  Product1 : Product  RndMeth=Zero
  Torque_Percentage : Outport
  wires:
  Nm_Torque/1 -> Divide1/1  "Nm_Torque"
  Product1/1 -> Torque_Percentage/1  "Torque_Percentage"
  Reference_Torque/1 -> Divide1/2  "Reference_Torque"
  Divide1/1 -> Product1/1
  Constant/1 -> Product1/2

== system Electrical_to_Mechanical_gen/EDB_DriveEmot/eMot 4 TX/Nm_to_percent3 ==
  Nm_Torque : Inport
  Reference_Torque : Inport  Port=2
  Constant : Constant  Value=100
  Divide1 : Product  Inputs=*/
  Product1 : Product  RndMeth=Zero
  Torque_Percentage : Outport
  wires:
  Constant/1 -> Product1/2
  Divide1/1 -> Product1/1
  Reference_Torque/1 -> Divide1/2  "Reference_Torque"
  Product1/1 -> Torque_Percentage/1  "Torque_Percentage"
  Nm_Torque/1 -> Divide1/1  "Nm_Torque"

== system Electrical_to_Mechanical_gen/e-Motor/Thermic_Model_Inverter/C_IGBT_and_Diode ==
  P_Heat_eff : Inport
  T : Inport  Port=2
  Add : Sum
  Digital Clock : DigitalClock  SampleTime=-1
  Divide : Product  Inputs=*/
  Heat_Capacity_PowerStack [J/K] : Constant  Value=drvEmot_inv_Cth_IGBT+drvEmot_inv_Cth_diode
  Product : Product
  Product1 : Product
  Sum : Sum  Inputs=|+-
  Unit Delay : UnitDelay  SampleTime=-1
  T_new : Outport
  wires:
  Sum/1 -> Product/2  "[s]"
  P_Heat_eff/1 -> Product/1
  Product/1 -> Add/1  "[J]"
  T/1 -> Product1/1  "[K]"
  Heat_Capacity_PowerStack [J/K]/1 -> Product1/2, Divide/2
  Product1/1 -> Add/2  "[J]"
  Add/1 -> Divide/1
  Divide/1 -> T_new/1  "[K]"
  Digital Clock/1 -> Sum/1, Unit Delay/1
  Unit Delay/1 -> Sum/2

== system Electrical_to_Mechanical_gen/e-Motor/Thermic_Model_Inverter/C_Plate ==
  P_Heat_eff : Inport
  T : Inport  Port=2
  Add : Sum
  Digital Clock : DigitalClock  SampleTime=-1
  Divide : Product  Inputs=*/
  Heat_Capacity_Plate [J/K] : Constant  Value=drvEmot_inv_Cth_cooling_plate
  Product : Product
  Product1 : Product
  Sum : Sum  Inputs=|+-
  Unit Delay : UnitDelay  SampleTime=-1
  T_new : Outport
  wires:
  Sum/1 -> Product/2  "[s]"
  P_Heat_eff/1 -> Product/1
  Product/1 -> Add/1  "[J]"
  T/1 -> Product1/1  "[K]"
  Product1/1 -> Add/2  "[J]"
  Add/1 -> Divide/1
  Divide/1 -> T_new/1  "[K]"
  Heat_Capacity_Plate [J/K]/1 -> Product1/2, Divide/2
  Digital Clock/1 -> Sum/1, Unit Delay/1
  Unit Delay/1 -> Sum/2

== system Electrical_to_Mechanical_gen/e-Motor/Thermic_Model_Inverter/R_PS-Plate ==
  T_IGBT : Inport
  T_Plate : Inport  Port=2
  Add : Sum  Inputs=+-
  Divide : Product  Inputs=*/
  R_th_IGBT_Plate : Constant  Value=drvEmot_inv_Rth_PS_cooling_plate
  dQ : Outport
  wires:
  R_th_IGBT_Plate/1 -> Divide/2
  Divide/1 -> dQ/1
  Add/1 -> Divide/1
  T_Plate/1 -> Add/2
  T_IGBT/1 -> Add/1

== system Electrical_to_Mechanical_gen/e-Motor/Thermic_Model_Inverter/R_Plate-Coolant ==
  T_Plate : Inport
  T_Coolant : Inport  Port=2
  Add : Sum  Inputs=+-
  Divide : Product  Inputs=*/
  Rth_cooling_plate_coolant : Constant  Value=drvEmot_inv_Rth_cooling_plate_coolant
  dQ : Outport
  wires:
  T_Plate/1 -> Add/1
  T_Coolant/1 -> Add/2
  Add/1 -> Divide/1
  Divide/1 -> dQ/1
  Rth_cooling_plate_coolant/1 -> Divide/2

== system Electrical_to_Mechanical_gen/e-Motor/Thermic_Model_PMSM_slot2/C_Rotor ==
  P_Heat_eff : Inport
  T : Inport  Port=2
  Add : Sum
  Digital Clock : DigitalClock  SampleTime=-1
  Divide : Product  Inputs=*/
  Heat_Capacity_Rotor [J/K] : Constant  Value=drvEmot_emot_Cth_rotor
  Product : Product
  Product1 : Product
  Sum : Sum  Inputs=|+-
  Unit Delay : UnitDelay  SampleTime=-1
  T_new : Outport
  wires:
  Divide/1 -> T_new/1  "[K]"
  Add/1 -> Divide/1
  Product1/1 -> Add/2  "[J]"
  Heat_Capacity_Rotor [J/K]/1 -> Divide/2, Product1/2
  T/1 -> Product1/1  "[K]"
  Product/1 -> Add/1  "[J]"
  P_Heat_eff/1 -> Product/1
  Sum/1 -> Product/2  "[s]"
  Digital Clock/1 -> Sum/1, Unit Delay/1
  Unit Delay/1 -> Sum/2

== system Electrical_to_Mechanical_gen/e-Motor/Thermic_Model_PMSM_slot2/C_Stator ==
  P_Heat_eff : Inport
  T : Inport  Port=2
  Add : Sum
  Digital Clock : DigitalClock  SampleTime=-1
  Divide : Product  Inputs=*/
  Heat_Capacity_Stator [J/K] : Constant  Value=drvEmot_emot_Cth_stator
  Product : Product
  Product1 : Product
  Sum : Sum  Inputs=|+-
  Unit Delay : UnitDelay  SampleTime=-1
  T_new : Outport
  wires:
  Sum/1 -> Product/2  "[s]"
  P_Heat_eff/1 -> Product/1
  Product/1 -> Add/1  "[J]"
  T/1 -> Product1/1  "[K]"
  Heat_Capacity_Stator [J/K]/1 -> Product1/2, Divide/2
  Product1/1 -> Add/2  "[J]"
  Add/1 -> Divide/1
  Divide/1 -> T_new/1  "[K]"
  Digital Clock/1 -> Sum/1, Unit Delay/1
  Unit Delay/1 -> Sum/2

== system Electrical_to_Mechanical_gen/e-Motor/Thermic_Model_PMSM_slot2/K2degC ==
  In1 : Inport
  Add : Sum  Inputs=+-
  Constant : Constant  Value=273.15
  Out1 : Outport
  wires:
  In1/1 -> Add/1
  Add/1 -> Out1/1
  Constant/1 -> Add/2

== system Electrical_to_Mechanical_gen/e-Motor/Thermic_Model_PMSM_slot2/K2degC1 ==
  In1 : Inport
  Add : Sum  Inputs=+-
  Constant : Constant  Value=273.15
  Out1 : Outport
  wires:
  In1/1 -> Add/1
  Add/1 -> Out1/1
  Constant/1 -> Add/2

== system Electrical_to_Mechanical_gen/e-Motor/Thermic_Model_PMSM_slot2/R_RotorOil ==
  T_Rotor : Inport
  T_Oil : Inport  Port=2
  Add : Sum  Inputs=+-
  Divide : Product  Inputs=*/
  R_th_Rot_Oil : Constant  Value=drvEmot_emot_Rth_rotor_oil
  dQ : Outport
  wires:
  T_Rotor/1 -> Add/1
  T_Oil/1 -> Add/2
  Add/1 -> Divide/1
  Divide/1 -> dQ/1
  R_th_Rot_Oil/1 -> Divide/2

== system Electrical_to_Mechanical_gen/e-Motor/Thermic_Model_PMSM_slot2/R_StatorOil ==
  T_Oil : Inport
  T_Stator : Inport  Port=2
  Add : Sum  Inputs=-+
  Divide : Product  Inputs=*/
  R_th_Stat_Oil : Constant  Value=drvEmot_emot_Rth_stator_oil
  dQ : Outport
  wires:
  T_Oil/1 -> Add/1
  T_Stator/1 -> Add/2
  Add/1 -> Divide/1
  Divide/1 -> dQ/1
  R_th_Stat_Oil/1 -> Divide/2

== system Electrical_to_Mechanical_gen/e-Motor/Thermic_Model_PMSM_slot2/R_StatorRotor ==
  T_Stator : Inport
  T_Rotor : Inport  Port=2
  Add : Sum  Inputs=+-
  Divide : Product  Inputs=*/
  R_th_Stat_Rot : Constant  Value=drvEmot_emot_Rth_stator_rotor
  dQ : Outport
  wires:
  R_th_Stat_Rot/1 -> Divide/2
  Divide/1 -> dQ/1
  Add/1 -> Divide/1
  T_Rotor/1 -> Add/2
  T_Stator/1 -> Add/1

== system Electrical_to_Mechanical_gen/e-Motor/Thermic_Model_PMSM_slot2/degC2K ==
  In1 : Inport
  Add : Sum
  Constant : Constant  Value=273.15
  Out1 : Outport
  wires:
  In1/1 -> Add/1
  Add/1 -> Out1/1
  Constant/1 -> Add/2

== system Electrical_to_Mechanical_gen/e-Motor/Thermic_Model_PMSM_slot2/degC2K1 ==
  In1 : Inport
  Add : Sum
  Constant : Constant  Value=273.15
  Out1 : Outport
  wires:
  Constant/1 -> Add/2
  Add/1 -> Out1/1
  In1/1 -> Add/1

== system Electrical_to_Mechanical_gen/e-Motor/Thermic_Model_PMSM_slot2/degC2K2 ==
  In1 : Inport
  Add : Sum
  Constant : Constant  Value=273.15
  Out1 : Outport
  wires:
  In1/1 -> Add/1
  Add/1 -> Out1/1
  Constant/1 -> Add/2

== matlab function Electrical_to_Mechanical_gen/EDB_DriveEmot/MotorSelection/Truth Table ==
  data: u1 input; y1 output; u2 input; y2 output; y3 output; y4 output
function [y1, y2, y3, y4] = fcn(u1, u2)

aVarTruthTableCondition_1 = false;
aVarTruthTableCondition_2 = false;
aVarTruthTableCondition_3 = false;
aVarTruthTableCondition_4 = false;
aVarTruthTableCondition_5 = false;
aVarTruthTableCondition_6 = false;
aVarTruthTableCondition_7 = false;
aVarTruthTableCondition_8 = false;
aVarTruthTableCondition_9 = false;


% 1stDrivenAxle - 0  and 2ndDrivenAxle - 0 [Not Valid]

aVarTruthTableCondition_1 = logical(u1 == 0 && u2 == 0);

% 1stDrivenAxle - 0  and 2ndDrivenAxle - 1 [Not Valid]

aVarTruthTableCondition_2 = logical(u1 == 0 && u2 == 1);

% 1stDrivenAxle - 0  and 2ndDrivenAxle - 2 [Not Valid]

aVarTruthTableCondition_3 = logical(u1 == 0 && u2 == 2);

% 1stDrivenAxle - 1  and 2ndDrivenAxle - 0 [Emot1,-]

aVarTruthTableCondition_4 = logical(u1 == 1 && u2 == 0);

% 1stDrivenAxle - 1  and 2ndDrivenAxle - 1 [Emot1, Emot3]

aVarTruthTableCondition_5 = logical(u1 == 1 && u2 == 1);

% 1stDrivenAxle - 1  and 2ndDrivenAxle - 2 [Emot1, Emot3+Emot4]

aVarTruthTableCondition_6 = logical(u1 == 1 && u2 == 2);

% 1stDrivenAxle - 2  and 2ndDrivenAxle - 0 [Emot1+Emot2,-]

aVarTruthTableCondition_7 = logical(u1 == 2 && u2 == 0);

% 1stDrivenAxle - 2  and 2ndDrivenAxle - 1 [Emot1+Emot2,Emot3]

aVarTruthTableCondition_8 = logical(u1 == 2 && u2 == 1);

% 1stDrivenAxle - 2  and2ndDrivenAxle - 2 [Emot1+Emot2,Emot3+Emot4]

aVarTruthTableCondition_9 = logical(u1 == 2 && u2 == 2);

if (aVarTruthTableCondition_1 && ~aVarTruthTableCondition_2 && ~aVarTruthTableCondition_3 && ~aVarTruthTableCondition_4 && ~aVarTruthTableCondition_5 && ~aVarTruthTableCondition_6 && ~aVarTruthTableCondition_7 && ~aVarTruthTableCondition_8 && ~aVarTruthTableCondition_9)
    aFcnTruthTableAction_1();
elseif (~aVarTruthTableCondition_1 && aVarTruthTableCondition_2 && ~aVarTruthTableCondition_3 && ~aVarTruthTableCondition_4 && ~aVarTruthTableCondition_5 && ~aVarTruthTableCondition_6 && ~aVarTruthTableCondition_7 && ~aVarTruthTableCondition_8 && ~aVarTruthTableCondition_9)
    aFcnTruthTableAction_2();
elseif (~aVarTruthTableCondition_1 && ~aVarTruthTableCondition_2 && aVarTruthTableCondition_3 && ~aVarTruthTableCondition_4 && ~aVarTruthTableCondition_5 && ~aVarTruthTableCondition_6 && ~aVarTruthTableCondition_7 && ~aVarTruthTableCondition_8 && ~aVarTruthTableCondition_9)
    aFcnTruthTableAction_3();
elseif (~aVarTruthTableCondition_1 && ~aVarTruthTableCondition_2 && ~aVarTruthTableCondition_3 && aVarTruthTableCondition_4 && ~aVarTruthTableCondition_5 && ~aVarTruthTableCondition_6 && ~aVarTruthTableCondition_7 && ~aVarTruthTableCondition_8 && ~aVarTruthTableCondition_9)
    aFcnTruthTableAction_4();
elseif (~aVarTruthTableCondition_1 && ~aVarTruthTableCondition_2 && ~aVarTruthTableCondition_3 && ~aVarTruthTableCondition_4 && aVarTruthTableCondition_5 && ~aVarTruthTableCondition_6 && ~aVarTruthTableCondition_7 && ~aVarTruthTableCondition_8 && ~aVarTruthTableCondition_9)
    aFcnTruthTableAction_5();
elseif (~aVarTruthTableCondition_1 && ~aVarTruthTableCondition_2 && ~aVarTruthTableCondition_3 && ~aVarTruthTableCondition_4 && ~aVarTruthTableCondition_5 && aVarTruthTableCondition_6 && ~aVarTruthTableCondition_7 && ~aVarTruthTableCondition_8 && ~aVarTruthTableCondition_9)
    aFcnTruthTableAction_6();
elseif (~aVarTruthTableCondition_1 && ~aVarTruthTableCondition_2 && ~aVarTruthTableCondition_3 && ~aVarTruthTableCondition_4 && ~aVarTruthTableCondition_5 && ~aVarTruthTableCondition_6 && aVarTruthTableCondition_7 && ~aVarTruthTableCondition_8 && ~aVarTruthTableCondition_9)
    aFcnTruthTableAction_7();
elseif (~aVarTruthTableCondition_1 && ~aVarTruthTableCondition_2 && ~aVarTruthTableCondition_3 && ~aVarTruthTableCondition_4 && ~aVarTruthTableCondition_5 && ~aVarTruthTableCondition_6 && ~aVarTruthTableCondition_7 && aVarTruthTableCondition_8 && ~aVarTruthTableCondition_9)
    aFcnTruthTableAction_8();
elseif (~aVarTruthTableCondition_1 && ~aVarTruthTableCondition_2 && ~aVarTruthTableCondition_3 && ~aVarTruthTableCondition_4 && ~aVarTruthTableCondition_5 && ~aVarTruthTableCondition_6 && ~aVarTruthTableCondition_7 && ~aVarTruthTableCondition_8 && aVarTruthTableCondition_9)
    aFcnTruthTableAction_9();
else % Default
    aFcnTruthTableAction_10();
end

function aFcnTruthTableAction_1()

% 1stDrivenAxle - 0 
% 2ndDrivenAxle - 0
% NOT VALID

y1 = 0;
y2 = 0;
y3 = 0;
y4 = 0;

function aFcnTruthTableAction_2()

% 1stDrivenAxle - 0 
% 2ndDrivenAxle - 1
% NOT VALID

y1 = 0;
y2 = 0;
y3 = 0;
y4 = 0;

function aFcnTruthTableAction_3()

% 1stDrivenAxle - 0 
% 2ndDrivenAxle - 2
% NOT VALID

y1 = 0;
y2 = 0;
y3 = 0;
y4 = 0;

function aFcnTruthTableAction_4()

% 1stDrivenAxle - 1 
% 2ndDrivenAxle - 0 [Emot1,-]

y1 = 1;
y2 = 0;
y3 = 0;
y4 = 0;

function aFcnTruthTableAction_5()

% 1stDrivenAxle - 1  
% 2ndDrivenAxle - 1 [Emot1, Emot3]

y1 = 1;
y2 = 0;
y3 = 1;
y4 = 0;

function aFcnTruthTableAction_6()

% 1stDrivenAxle - 1 
% 2ndDrivenAxle - 2 [Emot1, Emot3+Emot4]

y1 = 1;
y2 = 0;
y3 = 1;
y4 = 1;

function aFcnTruthTableAction_7()

% 1stDrivenAxle - 2  
% 2ndDrivenAxle - 0 [Emot1+Emot2,-]

y1 = 1;
y2 = 1;
y3 = 0;
y4 = 0;

function aFcnTruthTableAction_8()

% 1stDrivenAxle - 2  
% 2ndDrivenAxle - 1 [Emot1+Emot2,Emot3]

y1 = 1;
y2 = 1;
y3 = 1;
y4 = 0;

function aFcnTruthTableAction_9()

% 1stDrivenAxle - 2
% 2ndDrivenAxle - 2 [Emot1+Emot2,Emot3+Emot4]

y1 = 1;
y2 = 1;
y3 = 1;
y4 = 1;

function aFcnTruthTableAction_10()

% Default

y1 = 0;
y2 = 0;
y3 = 0;
y4 = 0;
